simulink model "practica_prbs"  (Simulink 5.0)
settings: Solver=ode45  StartTime=0.0  StopTime=100.0  FixedStep=.1  MaxStep=.1*ts  RelTol=1e-4
undefined symbols (not defined in the file): ts
settings Model: LastModifiedBy=-  ExtModeTrigMode=oneshot  ExtModeArmWhenConnect=off  LimitDataPoints=off  BlockReductionOpt=off  BooleanDataType=off

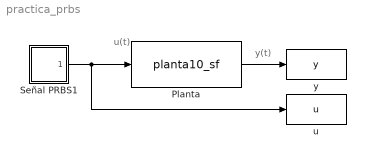
== system practica_prbs ==
  note: y(t)
  note: u(t)
  Planta : S-Function  FunctionName=planta10_sf  SFunctionModules=""  mask{rtw_sf_name=planta10_sf, showVar=off}
      mask prompts: rtw_sf_name "Generated S-function name (model_sf):"; showVar "Show module list"
      mask help: Real-Time Workshop generated S-function.
      mask init:
      | displist = '';
      | if ~strcmp(get_param(gcb, 'FunctionName'), rtw_sf_name);
      |   set_param(gcb, 'FunctionName', rtw_sf_name);
      | end
      | if  showVar & exist('rtwsfunc') == 2
      |   tmplist = rtwsfunc(rtw_sf_name,gcb);
      |   tmplist = ['\nList of Modules:\n', tmplist];
      | elseif showVar
      |   tmplist = '\nList of Modules:\nRTW not licensed\n';
      | end
      | if showVar
      |   displist = tmplist;
      | end
      settings: CopyFcn=set_param(gcb,'linkstatus','none')
      mask Help: web(['file://',docroot,'/toolbox/rtw/rtwsfcn.html']);
      mask Display:
      | port_label('input',1,'u(t)');
      | port_label('output',1,'y(t)');
  Señal PRBS1 : Subsystem
  u : ToWorkspace  VariableName=u  SampleTime=ts  SaveFormat=Array
  y : ToWorkspace  VariableName=y  SampleTime=ts  SaveFormat=Array
  wires:
  Señal PRBS1/1(u ( t )) -> u/1, Planta/1
  Planta/1 -> y/1

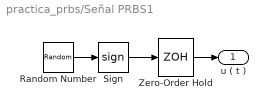
== system practica_prbs/Señal PRBS1 ==
  Random Number : RandomNumber  SampleTime=0
  Sign : Signum
  Zero-Order Hold : ZeroOrderHold  SampleTime=ts
  u ( t ) : Outport
  wires:
  Zero-Order Hold/1 -> u ( t )/1
  Sign/1 -> Zero-Order Hold/1
  Random Number/1 -> Sign/1
